simulink model "Model4"  (R2022a)
settings: Solver=VariableStepAuto  StartTime=0.0  StopTime=60  RelTol=1e-3  EnableMultiTasking=on
values from neighbouring files (symbols this model uses):
  A_actuator = 1    [Exam2018.m]
  Ac = [-2.5 0 0 ; 1 0 0 ; 0 1 0]    [Exam2018.m]
  Bc = [2.5 ; 0 ; 0]    [Exam2018.m]
  Cc = [0 0 1]    [Exam2018.m]
  K1c = Kc(1)    [Exam2018.m]
  K2c = Kc(2)    [Exam2018.m]
  K3c = Kc(3)    [Exam2018.m]
  L = place(Ac',Cc',random_fast_poles)'    [Exam2018.m]
  Nc = K3c    [Exam2018.m]
  tau = 0.4    [Exam2018.m]
settings Model: Creator=y.briere  LastModifiedBy=fades
settings SolverCC: AlgebraicLoopSolver=TrustRegion
settings DataIOCC: LimitDataPoints=on  ReturnWorkspaceOutputs=off
settings OptimizationCC: LifeSpan=inf
settings DebuggingCC: UnconnectedInputMsg=warning  UnconnectedOutputMsg=warning  UnconnectedLineMsg=warning  AllowSymbolicDim=off  SFUnexpectedBacktrackingDiag=warning  SFNoUnconditionalDefaultTransitionDiag=warning  SFExecutionAtInitializationDiag=none  SFMachineParentedDataDiag=warning  ArithmeticOperatorsInVariantConditions=warning
settings ModelReferenceCC: PropagateSignalLabelsOutOfModel=off
settings SFSimCC: SimUseLocalCustomCode=off  CustomCodeUndefinedFunction=UseInterfaceOnly
settings RTWCC: RTWUseLocalCustomCode=off
settings CodeAppCC: StateflowObjectComments=on
settings GRTTargetCC: TargetLangStandard=C89/C90 (ANSI)
settings ConfigComp: CovMetricSettings=dw  CovSaveCumulativeToWorkspaceVar=on  CovSaveSingleToWorkspaceVar=on  CovExternalEMLEnable=off

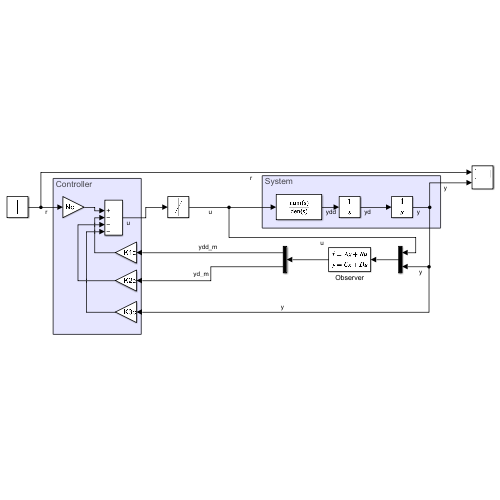
[thumbnail: Simulink's stored preview of the top-level diagram]
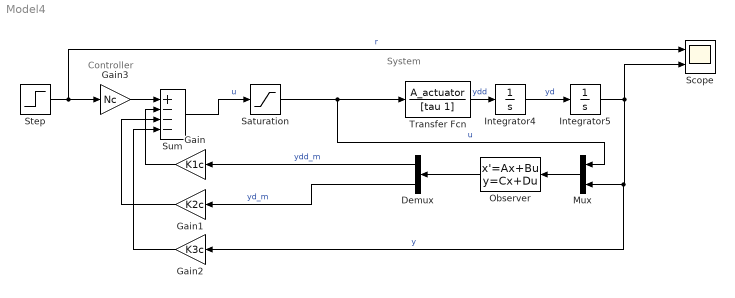
== system Model4 ==
  note: Controller
  note: System
  Demux : Demux  Outputs=2
  Gain : Gain  Gain=K1c
  Gain1 : Gain  Gain=K2c
  Gain2 : Gain  Gain=K3c
  Gain3 : Gain  Gain=Nc
  Integrator4 : Integrator
  Integrator5 : Integrator
  Mux : Mux  Inputs=2
  Observer : StateSpace  A=Ac-L*Cc  B=[Bc L]  C=[1 0 0 ; 0 1 0]  D=[0 0 ; 0 0]  InitialCondition=0
  Saturation : Saturate
  Scope : Scope  NumInputPorts=2
  Step : Step  SampleTime=0
  Sum : Sum  Inputs=|+---
  Transfer Fcn : TransferFcn  Numerator=A_actuator  Denominator=[tau 1]
  wires:
  Integrator4/1 -> Integrator5/1  "yd"
  Transfer Fcn/1 -> Integrator4/1  "ydd"
  Integrator5/1 -> Gain2/1, Mux/2, Scope/2  "y"
  Step/1 -> Scope/1, Gain3/1  "r"
  Gain3/1 -> Sum/1
  Mux/1 -> Observer/1
  Observer/1 -> Demux/1
  Demux/1 -> Gain/1  "ydd_m"
  Demux/2 -> Gain1/1  "yd_m"
  Sum/1 -> Saturation/1  "u"
  Saturation/1 -> Mux/1, Transfer Fcn/1  "u"
  Gain/1 -> Sum/2
  Gain1/1 -> Sum/3
  Gain2/1 -> Sum/4
